simulink model "two_area_model_3_phase"  (R2020a)
settings: Solver=VariableStepAuto  StartTime=0.0  StopTime=10.0  RelTol=1e-3
values from neighbouring files (symbols this model uses):
  ExpandSmachs = zeros(Nbus,NSmachs)    [Synch_parameter_gen_base.m]    (also in Synch_parameter_sys_base.m)
  s_D = mac_con(:,16)    [Synch_parameter_gen_base.m]    (also in Synch_parameter_sys_base.m = mac_con(:,16).*system_base_mva./machine_base_mva)
  s_delta = angle(s_Eq)    [generic_Sync_Init.m]
  s_Edd = -(s_xq - s_xqd).*s_iq    [generic_Sync_Init.m]
  s_Efd = abs(s_Eq)-(s_xd-s_xq).*s_id    [generic_Sync_Init.m]
  s_Eqd = s_Efd+ (s_xd - s_xdd).*s_id    [generic_Sync_Init.m]
  s_H = mac_con(:,15)    [Synch_parameter_gen_base.m]    (also in Synch_parameter_sys_base.m = mac_con(:,15).*system_base_mva./machine_base_mva)
  s_Ka = 200    [four_mac_data.m]    (also in two_area_synch.m)
  s_Psi2q = -s_Edd+(s_xqd - s_xls).*s_iq    [generic_Sync_Init.m]
  s_Rgov = s_Rgov    [Synch_parameter_gen_base.m]    (also in Synch_parameter_sys_base.m = s_Rgov.*system_base_mva./machine_base_mva; four_mac_data.m = 0.05; two_area_synch.m = 0.05)
  s_Rs = mac_con(:,4)    [Synch_parameter_gen_base.m]    (also in Synch_parameter_sys_base.m = mac_con(:,4).*system_base_mva./machine_base_mva)
  s_Ta = 0.02    [four_mac_data.m]    (also in two_area_synch.m)
  s_Tdod = mac_con(:,8)    [Synch_parameter_gen_base.m]    (also in Synch_parameter_sys_base.m)
  s_Tdodd = mac_con(:,9)    [Synch_parameter_gen_base.m]    (also in Synch_parameter_sys_base.m)
  s_Tg = 0.2    [four_mac_data.m]    (also in two_area_synch.m)
  s_Tm = s_Te    [generic_Sync_Init.m]
  s_Tqod = mac_con(:,13)    [Synch_parameter_gen_base.m]    (also in Synch_parameter_sys_base.m)
  s_Tqodd = mac_con(:,14)    [Synch_parameter_gen_base.m]    (also in Synch_parameter_sys_base.m)
  s_Vref = s_volt+1./s_Ka.*s_Efd    [generic_Sync_Init.m]
  s_ws = 1    [generic_Sync_Init.m]
  s_xd = mac_con(:,5)    [Synch_parameter_gen_base.m]    (also in Synch_parameter_sys_base.m = mac_con(:,5).*system_base_mva./machine_base_mva)
  s_xdd = mac_con(:,6)    [Synch_parameter_gen_base.m]    (also in Synch_parameter_sys_base.m = mac_con(:,6).*system_base_mva./machine_base_mva)
  s_xddd = mac_con(:,7)    [Synch_parameter_gen_base.m]    (also in Synch_parameter_sys_base.m = mac_con(:,7).*system_base_mva./machine_base_mva)
  s_xls = mac_con(:,3)    [Synch_parameter_gen_base.m]    (also in Synch_parameter_sys_base.m = mac_con(:,3).*system_base_mva./machine_base_mva)
  s_xq = mac_con(:,10)    [Synch_parameter_gen_base.m]    (also in Synch_parameter_sys_base.m = mac_con(:,10).*system_base_mva./machine_base_mva)
  s_xqd = mac_con(:,11)    [Synch_parameter_gen_base.m]    (also in Synch_parameter_sys_base.m = mac_con(:,11).*system_base_mva./machine_base_mva)
  s_xqdd = mac_con(:,12)    [Synch_parameter_gen_base.m]    (also in Synch_parameter_sys_base.m = mac_con(:,12).*system_base_mva./machine_base_mva)
  SelectSmachs = zeros(NSmachs,Nbus)    [Synch_parameter_gen_base.m]    (also in Synch_parameter_sys_base.m)
  Z = inv(Y)    [four_mac_data.m]    (also in four_mac_run.m; two_area_synch.m)
  zf = inv(Yf)    [four_mac_run.m]    (also in two_area_synch.m)
undefined symbols (not defined in the file or in its folder): j, s_Psild
settings Model: Creator=lenovo  LastModifiedBy=EBUKA
settings OptimizationCC: LifeSpan=inf
settings DebuggingCC: ArithmeticOperatorsInVariantConditions=warning
settings SFSimCC: CustomCodeUndefinedFunction=UseInterfaceOnly
settings CodeAppCC: StateflowObjectComments=on
settings SimscapeCC: SimscapeNormalizeSystem=off

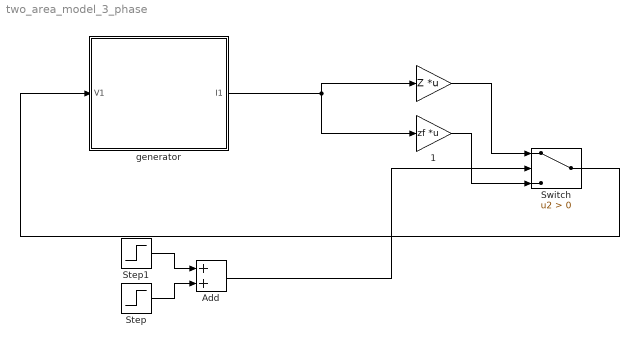
== system two_area_model_3_phase ==
  "       " : Gain  Gain=Z  Multiplication=Matrix(K*u)
  "       1" : Gain  Gain=zf  Multiplication=Matrix(K*u)
  Add : Sum
  Step : Step  Before=1  After=1.1  SampleTime=0
  Step1 : Step  Before=1  After=1.1  SampleTime=0
  Switch : Switch  Criteria=u2 > Threshold
  generator : Subsystem
  wires:
  "       1"/1 -> Switch/3
  Switch/1 -> generator/1(V1)
  "       "/1 -> Switch/1
  generator/1(I1) -> "       1"/1, "       "/1
  Step1/1 -> Add/1
  Step/1 -> Add/2
  Add/1 -> Switch/2

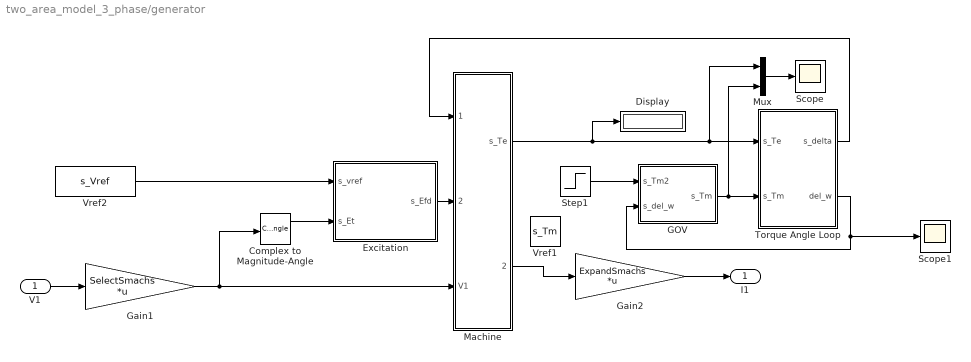
== system two_area_model_3_phase/generator ==
  V1 : Inport
  Complex to Magnitude-Angle : ComplexToMagnitudeAngle
  Display : Display
  Excitation : Subsystem
  GOV : Subsystem
  Gain1 : Gain  Gain=SelectSmachs  Multiplication=Matrix(K*u)
  Gain2 : Gain  Gain=ExpandSmachs  Multiplication=Matrix(K*u)
  Machine : Subsystem
  Mux : Mux  Inputs=2
  Scope : Scope
  Scope1 : Scope
  Step1 : Step  Time=2  Before=s_Tm  After=s_Tm+0.07031  SampleTime=0
  Torque Angle Loop : Subsystem
  Vref1 : Constant  Value=s_Tm
  Vref2 : Constant  Value=s_Vref
  I1 : Outport
  wires:
  V1/1 -> Gain1/1
  Gain2/1 -> I1/1
  Torque Angle Loop/1(s_delta) -> Machine/1(s_delta)
  Machine/1(s_Te) -> Display/1, Torque Angle Loop/1("s_Te "), Mux/1
  Machine/2(s_iDQ) -> Gain2/1
  Torque Angle Loop/2(del_w) -> Scope1/1, GOV/2(s_del_w)
  Complex to Magnitude-Angle/1 -> Excitation/2(s_Et)
  Mux/1 -> Scope/1
  GOV/1(s_Tm) -> Mux/2, Torque Angle Loop/2(s_Tm)
  Vref2/1 -> Excitation/1(s_vref)
  Step1/1 -> GOV/1(s_Tm2)
  Excitation/1(s_Efd) -> Machine/2(s_Efd)
  Gain1/1 -> Machine/3(V1), Complex to Magnitude-Angle/1

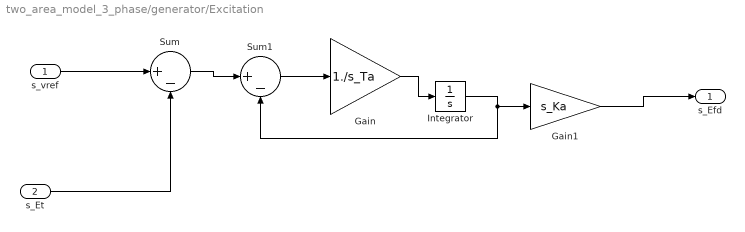
== system two_area_model_3_phase/generator/Excitation ==
  s_vref : Inport
  s_Et : Inport  Port=2
  Gain : Gain  Gain=1./s_Ta
  Gain1 : Gain  Gain=s_Ka
  Integrator : Integrator  InitialCondition=s_Efd./s_Ka
  Sum : Sum  Inputs=|+-
  Sum1 : Sum  Inputs=|+-
  s_Efd : Outport
  wires:
  Sum1/1 -> Gain/1
  Sum/1 -> Sum1/1
  Gain/1 -> Integrator/1
  Integrator/1 -> Sum1/2, Gain1/1
  Gain1/1 -> s_Efd/1
  s_vref/1 -> Sum/1
  s_Et/1 -> Sum/2

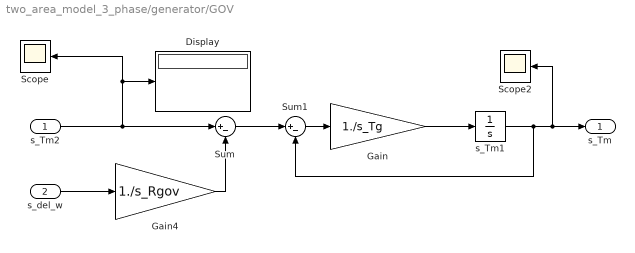
== system two_area_model_3_phase/generator/GOV ==
  s_Tm2 : Inport
  s_del_w : Inport  Port=2
  Display : Display
  Gain : Gain  Gain=1./s_Tg
  Gain4 : Gain  Gain=1./s_Rgov
  Scope : Scope
  Scope2 : Scope
  Sum : Sum  Inputs=|+-
  Sum1 : Sum  Inputs=|+-
  s_Tm1 : Integrator  InitialCondition=s_Tm
  s_Tm : Outport
  wires:
  s_Tm2/1 -> Scope/1, Display/1, Sum/1
  s_del_w/1 -> Gain4/1
  Gain4/1 -> Sum/2
  Sum/1 -> Sum1/1
  Sum1/1 -> Gain/1
  Gain/1 -> s_Tm1/1
  s_Tm1/1 -> Sum1/2, Scope2/1, s_Tm/1

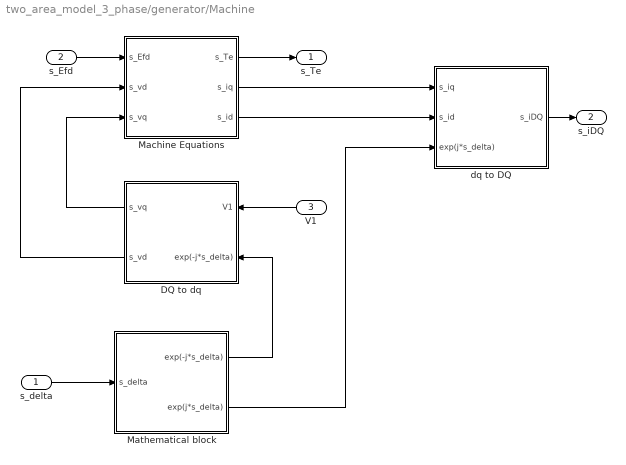
== system two_area_model_3_phase/generator/Machine ==
  s_delta : Inport
  s_Efd : Inport  Port=2
  V1 : Inport  Port=3
  DQ to dq : Subsystem
  Machine Equations : Subsystem
  Mathematical block : Subsystem
  dq to DQ : Subsystem
  s_Te : Outport
  s_iDQ : Outport  Port=2
  wires:
  s_Efd/1 -> Machine Equations/1(s_Efd)
  Machine Equations/1(s_Te) -> s_Te/1
  Machine Equations/2(s_iq) -> dq to DQ/1(s_iq)
  Machine Equations/3(s_id) -> dq to DQ/2(s_id)
  V1/1 -> DQ to dq/1(V1)
  DQ to dq/1("s_vq ") -> Machine Equations/3(s_vq)
  DQ to dq/2(s_vd) -> Machine Equations/2(s_vd)
  s_delta/1 -> Mathematical block/1(s_delta)
  Mathematical block/1(exp(-j*s_delta)) -> DQ to dq/2(exp(-j*s_delta))
  Mathematical block/2(exp(j*s_delta)) -> dq to DQ/3(exp(j*s_delta))
  dq to DQ/1(s_iDQ) -> s_iDQ/1

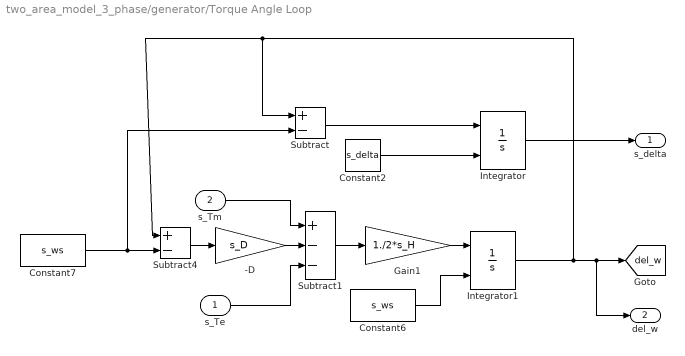
== system two_area_model_3_phase/generator/Torque Angle Loop ==
  "s_Te " : Inport
  s_Tm : Inport  Port=2
  -D : Gain  Gain=s_D
  Constant2 : Constant  Value=s_delta  VectorParams1D=off
  Constant6 : Constant  Value=s_ws  VectorParams1D=off
  Constant7 : Constant  Value=s_ws  VectorParams1D=off
  Gain1 : Gain  Gain=1./2*s_H
  Integrator : Integrator  InitialConditionSource=external
  Integrator1 : Integrator  InitialConditionSource=external
  Subtract : Sum  Inputs=+-
  Subtract1 : Sum  Inputs=+--
  Subtract4 : Sum  Inputs=+-
  s_delta : Outport
  del_w : Outport  Port=2
  tag scope: del_w=global
  wires:
  Subtract/1 -> Integrator/1
  s_Tm/1 -> Subtract1/1
  Subtract1/1 -> Gain1/1
  Gain1/1 -> Integrator1/1
  Constant6/1 -> Integrator1/2
  -D/1 -> Subtract1/2
  "s_Te "/1 -> Subtract1/3
  Integrator/1 -> s_delta/1
  Subtract4/1 -> -D/1
  Constant7/1 -> Subtract/2, Subtract4/2
  Constant2/1 -> Integrator/2
  Integrator1/1 -> Subtract/1, Subtract4/1, del_w/1, [del_w]

== system two_area_model_3_phase/generator/Machine/DQ to dq ==
  V1 : Inport
  exp(-j*s_delta) : Inport  Port=2
  Complex to Real-Imag : ComplexToRealImag
  Product1 : Product
  "s_vq " : Outport
  s_vd : Outport  Port=2
  wires:
  Complex to Real-Imag/1 -> "s_vq "/1
  Complex to Real-Imag/2 -> s_vd/1
  Product1/1 -> Complex to Real-Imag/1
  V1/1 -> Product1/1
  exp(-j*s_delta)/1 -> Product1/2

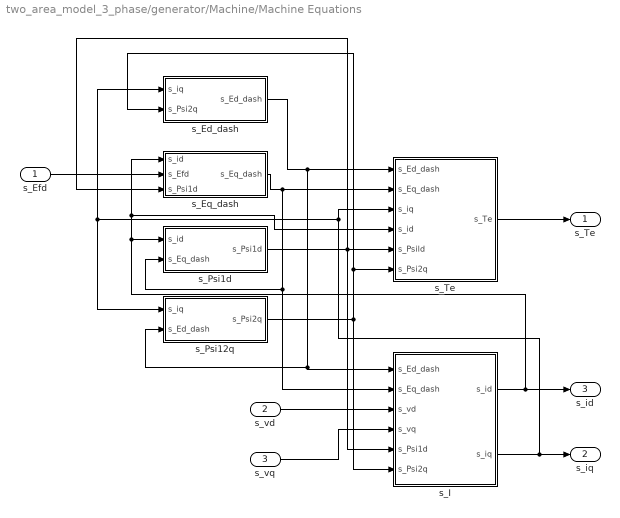
== system two_area_model_3_phase/generator/Machine/Machine Equations ==
  s_Efd : Inport
  s_vd : Inport  Port=2
  s_vq : Inport  Port=3
  s_Ed_dash : Subsystem
  s_Eq_dash : Subsystem
  s_I : Subsystem
  s_Psi12q : Subsystem
  s_Psi1d : Subsystem
  "s_Te " : Subsystem
  s_Te : Outport
  s_iq : Outport  Port=2
  s_id : Outport  Port=3
  wires:
  "s_Te "/1(s_Te) -> s_Te/1
  s_Efd/1 -> s_Eq_dash/2(s_Efd)
  s_Eq_dash/1(s_Eq_dash) -> s_Psi1d/2(s_Eq_dash), s_I/2(s_Eq_dash), "s_Te "/2(s_Eq_dash)
  s_I/1(s_id) -> s_Psi1d/1(s_id), "s_Te "/4(s_id), s_Eq_dash/1(s_id), s_id/1
  s_I/2(s_iq) -> "s_Te "/3(s_iq), s_Ed_dash/1(s_iq), s_Psi12q/1(s_iq), s_iq/1
  s_vd/1 -> s_I/3(s_vd)
  s_vq/1 -> s_I/4(s_vq)
  s_Ed_dash/1(s_Ed_dash) -> s_Psi12q/2(s_Ed_dash), s_I/1(s_Ed_dash), "s_Te "/1(s_Ed_dash)
  s_Psi12q/1(s_Psi2q) -> s_I/6(s_Psi2q), "s_Te "/6(s_Psi2q), s_Ed_dash/2(s_Psi2q)
  s_Psi1d/1(s_Psi1d) -> s_I/5(s_Psi1d), s_Eq_dash/3(s_Psi1d), "s_Te "/5(s_Psild)

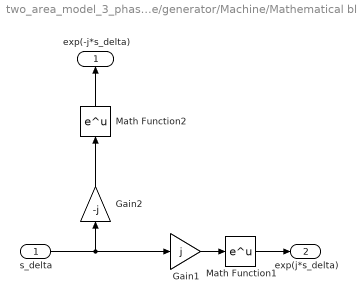
== system two_area_model_3_phase/generator/Machine/Mathematical block ==
  s_delta : Inport
  Gain1 : Gain  Gain=j
  Gain2 : Gain  Gain=-j
  Math Function1 : Math  SignedPower=on  SaturateOnIntegerOverflow=on
  Math Function2 : Math  SignedPower=on  SaturateOnIntegerOverflow=on
  exp(-j*s_delta) : Outport
  exp(j*s_delta) : Outport  Port=2
  wires:
  Gain1/1 -> Math Function1/1
  Gain2/1 -> Math Function2/1
  Math Function1/1 -> exp(j*s_delta)/1
  s_delta/1 -> Gain2/1, Gain1/1
  Math Function2/1 -> exp(-j*s_delta)/1

== system two_area_model_3_phase/generator/Machine/dq to DQ ==
  s_iq : Inport
  s_id : Inport  Port=2
  exp(j*s_delta) : Inport  Port=3
  Product : Product
  Real-Imag to Complex : RealImagToComplex
  s_iDQ : Outport
  wires:
  s_iq/1 -> Real-Imag to Complex/1
  s_id/1 -> Real-Imag to Complex/2
  Real-Imag to Complex/1 -> Product/1
  Product/1 -> s_iDQ/1
  exp(j*s_delta)/1 -> Product/2

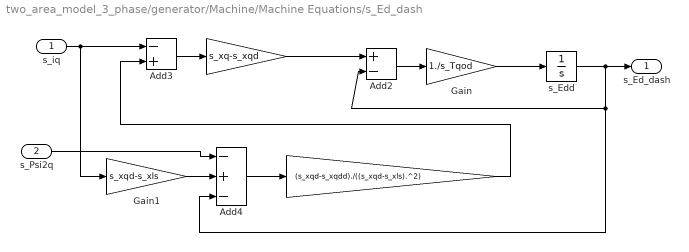
== system two_area_model_3_phase/generator/Machine/Machine Equations/s_Ed_dash ==
  s_iq : Inport
  s_Psi2q : Inport  Port=2
  " " : Gain  Gain=s_xq-s_xqd
  "  " : Gain  Gain=(s_xqd-s_xqdd)./((s_xqd-s_xls).^2)
  Add2 : Sum  Inputs=+-
  Add3 : Sum  Inputs=-+
  Add4 : Sum  Inputs=-+-
  Gain : Gain  Gain=1./s_Tqod
  Gain1 : Gain  Gain=s_xqd-s_xls
  s_Edd : Integrator  InitialCondition=s_Edd
  s_Ed_dash : Outport
  wires:
  s_iq/1 -> Gain1/1, Add3/1
  Add3/1 -> " "/1
  " "/1 -> Add2/1
  Gain1/1 -> Add4/2
  s_Psi2q/1 -> Add4/1
  Add2/1 -> Gain/1
  Gain/1 -> s_Edd/1
  s_Edd/1 -> Add2/2, Add4/3, s_Ed_dash/1
  Add4/1 -> "  "/1
  "  "/1 -> Add3/2

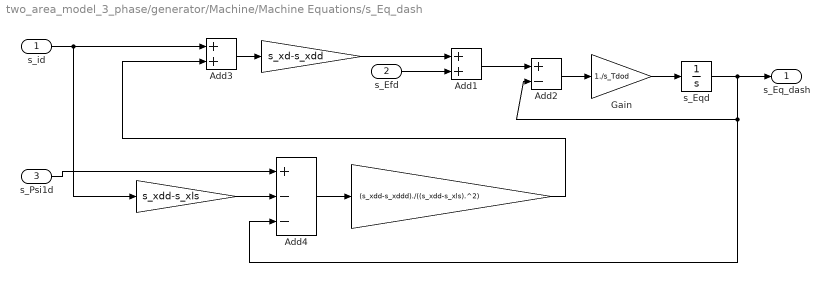
== system two_area_model_3_phase/generator/Machine/Machine Equations/s_Eq_dash ==
  s_id : Inport
  s_Efd : Inport  Port=2
  s_Psi1d : Inport  Port=3
  "  " : Gain  Gain=s_xdd-s_xls
  "    " : Gain  Gain=s_xd-s_xdd
  "         " : Gain  Gain=(s_xdd-s_xddd)./((s_xdd-s_xls).^2)
  Add1 : Sum
  Add2 : Sum  Inputs=+-
  Add3 : Sum
  Add4 : Sum  Inputs=+--
  Gain : Gain  Gain=1./s_Tdod
  s_Eqd : Integrator  InitialCondition=s_Eqd
  s_Eq_dash : Outport
  wires:
  s_id/1 -> "  "/1, Add3/1
  Add3/1 -> "    "/1
  "  "/1 -> Add4/2
  s_Psi1d/1 -> Add4/1
  "    "/1 -> Add1/1
  s_Efd/1 -> Add1/2
  Add4/1 -> "         "/1
  "         "/1 -> Add3/2
  Add1/1 -> Add2/1
  Add2/1 -> Gain/1
  Gain/1 -> s_Eqd/1
  s_Eqd/1 -> Add2/2, Add4/3, s_Eq_dash/1

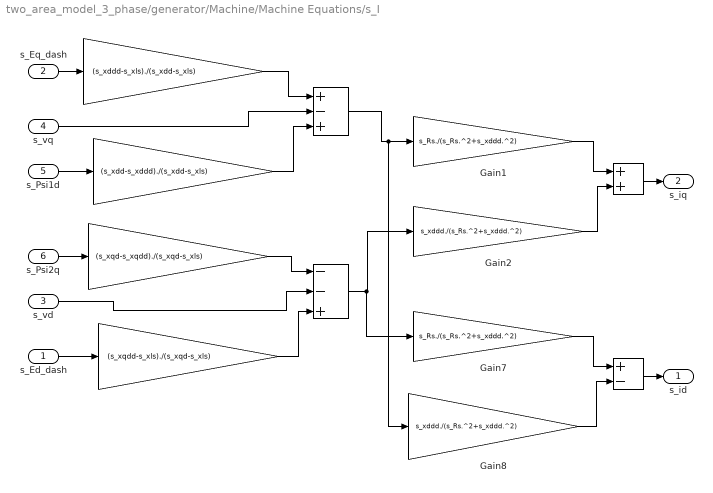
== system two_area_model_3_phase/generator/Machine/Machine Equations/s_I ==
  s_Ed_dash : Inport
  s_Eq_dash : Inport  Port=2
  s_vd : Inport  Port=3
  s_vq : Inport  Port=4
  s_Psi1d : Inport  Port=5
  s_Psi2q : Inport  Port=6
  " " : Sum  Inputs=+-+
  "  " : Gain  Gain=(s_xddd-s_xls)./(s_xdd-s_xls)
  "   " : Gain  Gain=(s_xdd-s_xddd)./(s_xdd-s_xls)
  "    " : Gain  Gain=(s_xqd-s_xqdd)./(s_xqd-s_xls)
  "      " : Sum  Inputs=--+
  "       " : Gain  Gain=(s_xqdd-s_xls)./(s_xqd-s_xls)
  "         " : Sum
  "            " : Sum  Inputs=+-
  Gain1 : Gain  Gain=s_Rs./(s_Rs.^2+s_xddd.^2)
  Gain2 : Gain  Gain=s_xddd./(s_Rs.^2+s_xddd.^2)
  Gain7 : Gain  Gain=s_Rs./(s_Rs.^2+s_xddd.^2)
  Gain8 : Gain  Gain=s_xddd./(s_Rs.^2+s_xddd.^2)
  s_id : Outport
  s_iq : Outport  Port=2
  wires:
  s_Eq_dash/1 -> "  "/1
  s_Psi1d/1 -> "   "/1
  s_vq/1 -> " "/2
  "  "/1 -> " "/1
  "   "/1 -> " "/3
  s_Psi2q/1 -> "    "/1
  "       "/1 -> "      "/3
  s_vd/1 -> "      "/2
  s_Ed_dash/1 -> "       "/1
  " "/1 -> Gain8/1, Gain1/1
  "      "/1 -> Gain7/1, Gain2/1
  Gain1/1 -> "         "/1
  Gain2/1 -> "         "/2
  Gain7/1 -> "            "/1
  Gain8/1 -> "            "/2
  "         "/1 -> s_iq/1
  "            "/1 -> s_id/1
  "    "/1 -> "      "/1

== system two_area_model_3_phase/generator/Machine/Machine Equations/s_Psi12q ==
  s_iq : Inport
  s_Ed_dash : Inport  Port=2
  " " : Gain  Gain=s_xqd-s_xls
  " Gain" : Gain  Gain=1./s_Tqodd
  Add2 : Sum  Inputs=+--
  s_Psi2_q : Integrator  InitialCondition=s_Psi2q
  s_Psi2q : Outport
  wires:
  s_iq/1 -> " "/1
  " "/1 -> Add2/1
  s_Ed_dash/1 -> Add2/2
  Add2/1 -> " Gain"/1
  " Gain"/1 -> s_Psi2_q/1
  s_Psi2_q/1 -> Add2/3, s_Psi2q/1

== system two_area_model_3_phase/generator/Machine/Machine Equations/s_Psi1d ==
  s_id : Inport
  s_Eq_dash : Inport  Port=2
  " " : Gain  Gain=s_xdd-s_xls
  Add2 : Sum  Inputs=++-
  Gain : Gain  Gain=1./s_Tdodd
  s_Psi1_d : Integrator  InitialCondition=s_Psild
  s_Psi1d : Outport
  wires:
  s_id/1 -> " "/1
  " "/1 -> Add2/1
  s_Eq_dash/1 -> Add2/2
  Add2/1 -> Gain/1
  Gain/1 -> s_Psi1_d/1
  s_Psi1_d/1 -> Add2/3, s_Psi1d/1

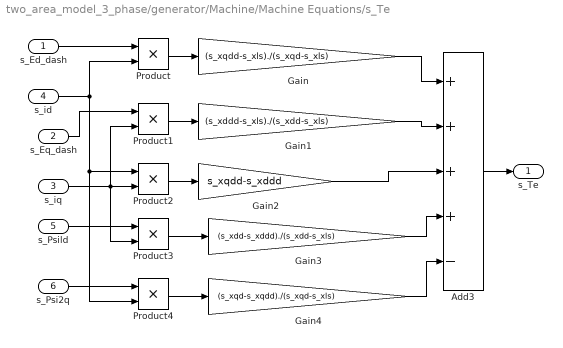
== system two_area_model_3_phase/generator/Machine/Machine Equations/s_Te  ==
  s_Ed_dash : Inport
  s_Eq_dash : Inport  Port=2
  s_iq : Inport  Port=3
  s_id : Inport  Port=4
  s_Psild : Inport  Port=5
  s_Psi2q : Inport  Port=6
  Add3 : Sum  Inputs=++++-
  Gain : Gain  Gain=(s_xqdd-s_xls)./(s_xqd-s_xls)
  Gain1 : Gain  Gain=(s_xddd-s_xls)./(s_xdd-s_xls)
  Gain2 : Gain  Gain=s_xqdd-s_xddd
  Gain3 : Gain  Gain=(s_xdd-s_xddd)./(s_xdd-s_xls)
  Gain4 : Gain  Gain=(s_xqd-s_xqdd)./(s_xqd-s_xls)
  Product{,1..4} (5 alike) : Product
  s_Te : Outport
  wires:
  s_Ed_dash/1 -> Product/1
  Product/1 -> Gain/1
  Product1/1 -> Gain1/1
  Product2/1 -> Gain2/1
  Product3/1 -> Gain3/1
  Product4/1 -> Gain4/1
  Gain/1 -> Add3/1
  Gain1/1 -> Add3/2
  Gain2/1 -> Add3/3
  Gain3/1 -> Add3/4
  Gain4/1 -> Add3/5
  s_Psi2q/1 -> Product4/1
  s_Psild/1 -> Product3/1
  s_iq/1 -> Product3/2, Product1/2, Product2/2
  s_Eq_dash/1 -> Product1/1
  s_id/1 -> Product/2, Product4/2, Product2/1
  Add3/1 -> s_Te/1
